simulink model "Numerical_Analysis_Final_Model"  (R2013a)
settings: Solver=ode4  StartTime=Tstart  StopTime=Tfinal  FixedStep=Ts  RelTol=1e-3
values from neighbouring files (symbols this model uses):
  Kd = 0.003    [Numerical_Analysis_Final.m]
  Kp = 27    [Numerical_Analysis_Final.m]
  Ldelta = 16000    [Numerical_Analysis_Final.m]
  Lp = 3.2    [Numerical_Analysis_Final.m]
  Lphi = 1200    [Numerical_Analysis_Final.m]
  phi_c = phi_cs(j)    [Numerical_Analysis_Final.m]
  phi_initial = phi_c + pi/180    [Numerical_Analysis_Final.m]
  Wa = Was(i)    [Numerical_Analysis_Final.m]
  Ws = 2*pi*100    (= 628.318530718)    [Numerical_Analysis_Final.m]
  zetaA = 0.7    [Numerical_Analysis_Final.m]
  zetaS = 0.7    [Numerical_Analysis_Final.m]
settings Model: Creator=Administrator  LastModifiedBy=Administrator
settings DataIOCC: LimitDataPoints=off

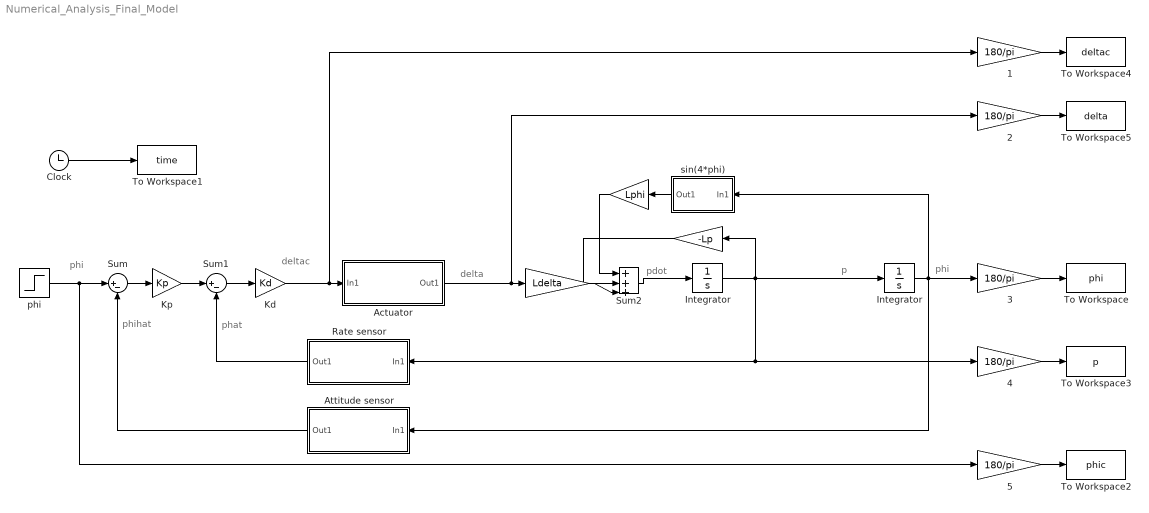
== system Numerical_Analysis_Final_Model ==
  note: phi
  note: phat
  note: phihat
  note: phi
  note: deltac
  note: delta
  note: pdot
  note: p
  "  " : Gain  Gain=Lphi
  "   " : Gain  Gain=Ldelta
  "           " : Gain  Gain=-Lp
     {1..5} (5 alike) : Gain  Gain=180/pi
  Actuator : Subsystem
  Attitude sensor : Subsystem
  Clock : Clock
  Integrator : Integrator  InitialCondition=phi_initial
  "Integrator " : Integrator
  Kd : Gain  Gain=Kd
  Kp : Gain  Gain=Kp
  Rate sensor : Subsystem
  Sum : Sum  Inputs=|+-
  Sum1 : Sum  Inputs=|+-
  Sum2 : Sum  Inputs=|+++
  To Workspace : ToWorkspace  VariableName=phi  SampleTime=-1
  To Workspace1 : ToWorkspace  VariableName=time  SampleTime=-1
  To Workspace2 : ToWorkspace  VariableName=phic  SampleTime=-1
  To Workspace3 : ToWorkspace  VariableName=p  SampleTime=-1
  To Workspace4 : ToWorkspace  VariableName=deltac  SampleTime=-1
  To Workspace5 : ToWorkspace  VariableName=delta  SampleTime=-1
  phi : Step  Time=0  After=phi_c  SampleTime=0
  sin(4*phi) : Subsystem
  wires:
  Sum/1 -> Kp/1
  Kp/1 -> Sum1/1
  Sum1/1 -> Kd/1
  Kd/1 -> "   1"/1, Actuator/1(In1)
  Clock/1 -> To Workspace1/1
  Attitude sensor/1(Out1) -> Sum/2
  Rate sensor/1(Out1) -> Sum1/2
  Actuator/1(Out1) -> "   "/1, "   2"/1
  sin(4*phi)/1(Out1) -> "  "/1
  "   "/1 -> Sum2/3
  "           "/1 -> Sum2/2
  "  "/1 -> Sum2/1
  Integrator/1 -> sin(4*phi)/1(In1), "   3"/1, Attitude sensor/1(In1)
  phi/1 -> "   5"/1, Sum/1
  Sum2/1 -> "Integrator "/1
  "Integrator "/1 -> "   4"/1, Rate sensor/1(In1), "           "/1, Integrator/1
  "   1"/1 -> To Workspace4/1
  "   2"/1 -> To Workspace5/1
  "   3"/1 -> To Workspace/1
  "   4"/1 -> To Workspace3/1
  "   5"/1 -> To Workspace2/1

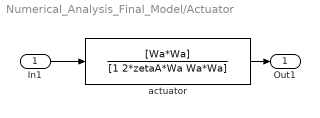
== system Numerical_Analysis_Final_Model/Actuator ==
  In1 : Inport
  actuator : TransferFcn  Numerator=[Wa*Wa]  Denominator=[1 2*zetaA*Wa Wa*Wa]
  Out1 : Outport
  wires:
  In1/1 -> actuator/1
  actuator/1 -> Out1/1

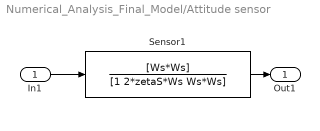
== system Numerical_Analysis_Final_Model/Attitude sensor ==
  In1 : Inport
  Sensor1 : TransferFcn  Numerator=[Ws*Ws]  Denominator=[1 2*zetaS*Ws Ws*Ws]
  Out1 : Outport
  wires:
  In1/1 -> Sensor1/1
  Sensor1/1 -> Out1/1

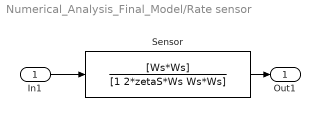
== system Numerical_Analysis_Final_Model/Rate sensor ==
  In1 : Inport
  Sensor : TransferFcn  Numerator=[Ws*Ws]  Denominator=[1 2*zetaS*Ws Ws*Ws]
  Out1 : Outport
  wires:
  In1/1 -> Sensor/1
  Sensor/1 -> Out1/1

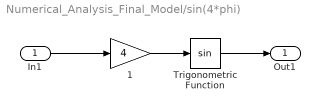
== system Numerical_Analysis_Final_Model/sin(4*phi) ==
  In1 : Inport
  " 1" : Gain  Gain=4
  Trigonometric Function : Trigonometry
  Out1 : Outport
  wires:
  In1/1 -> " 1"/1
  Trigonometric Function/1 -> Out1/1
  " 1"/1 -> Trigonometric Function/1
